simulink model "ConstantEnum"  (R2017b)
settings: Solver=FixedStepDiscrete  StartTime=0.0  StopTime=10.0  FixedStep=1.000000  RelTol=1e-3
model workspace (MAT data in the model file):
  ContractValidatorBlocksMap = containers.Map
  ContractValidatorBlocksMap.serialization.keys = {'DaysEnum/contract/validator', 'days/contract/validator'}
  ContractValidatorBlocksMap.serialization.values{1}.block = 'DaysEnum/contract/validator'
  ContractValidatorBlocksMap.serialization.values{1}.assumePorts = 0
  ContractValidatorBlocksMap.serialization.values{1}.guaranteePorts = 1
  ContractValidatorBlocksMap.serialization.values{1}.modeBlocksPorts = 0
  ContractValidatorBlocksMap.serialization.values{1}.portHandles.Inport = 64.0010986328
  ContractValidatorBlocksMap.serialization.values{1}.portHandles.Outport = 65.0003662109
  ContractValidatorBlocksMap.serialization.values{1}.portHandles.Enable = []
  ContractValidatorBlocksMap.serialization.values{1}.portHandles.Trigger = []
  ContractValidatorBlocksMap.serialization.values{1}.portHandles.State = []
  ContractValidatorBlocksMap.serialization.values{1}.portHandles.LConn = []
  ContractValidatorBlocksMap.serialization.values{1}.portHandles.RConn = []
  ContractValidatorBlocksMap.serialization.values{1}.portHandles.Ifaction = []
  ContractValidatorBlocksMap.serialization.values{1}.portHandles.Reset = []
  ContractValidatorBlocksMap.serialization.values{1}.portConnectivity(1).Type = '1'
  ContractValidatorBlocksMap.serialization.values{1}.portConnectivity(1).Position = [375 75]
  ContractValidatorBlocksMap.serialization.values{1}.portConnectivity(1).SrcBlock = 10.0003662109
  ContractValidatorBlocksMap.serialization.values{1}.portConnectivity(1).SrcPort = 0
  ContractValidatorBlocksMap.serialization.values{1}.portConnectivity(1).DstBlock = []
  ContractValidatorBlocksMap.serialization.values{1}.portConnectivity(1).DstPort = []
  ContractValidatorBlocksMap.serialization.values{1}.portConnectivity(2).Type = '1'
  ContractValidatorBlocksMap.serialization.values{1}.portConnectivity(2).Position = [505 75]
  ContractValidatorBlocksMap.serialization.values{1}.portConnectivity(2).SrcBlock = []
  ContractValidatorBlocksMap.serialization.values{1}.portConnectivity(2).SrcPort = []
  ContractValidatorBlocksMap.serialization.values{1}.portConnectivity(2).DstBlock = 35.0003662109
  ContractValidatorBlocksMap.serialization.values{1}.portConnectivity(2).DstPort = 0
  ContractValidatorBlocksMap.serialization.values{2}.block = 'days/contract/validator'
  ContractValidatorBlocksMap.serialization.values{2}.assumePorts = 0
  ContractValidatorBlocksMap.serialization.values{2}.guaranteePorts = 1
  ContractValidatorBlocksMap.serialization.values{2}.modeBlocksPorts = 0
  ContractValidatorBlocksMap.serialization.values{2}.portHandles.Inport = 174.00012207
  ContractValidatorBlocksMap.serialization.values{2}.portHandles.Outport = 168.000366211
  ContractValidatorBlocksMap.serialization.values{2}.portHandles.Enable = []
  ContractValidatorBlocksMap.serialization.values{2}.portHandles.Trigger = []
  ContractValidatorBlocksMap.serialization.values{2}.portHandles.State = []
  ContractValidatorBlocksMap.serialization.values{2}.portHandles.LConn = []
  ContractValidatorBlocksMap.serialization.values{2}.portHandles.RConn = []
  ContractValidatorBlocksMap.serialization.values{2}.portHandles.Ifaction = []
  ContractValidatorBlocksMap.serialization.values{2}.portHandles.Reset = []
  ContractValidatorBlocksMap.serialization.values{2}.portConnectivity(1).Type = '1'
  ContractValidatorBlocksMap.serialization.values{2}.portConnectivity(1).Position = [375 75]
  ContractValidatorBlocksMap.serialization.values{2}.portConnectivity(1).SrcBlock = 290.00012207
  ContractValidatorBlocksMap.serialization.values{2}.portConnectivity(1).SrcPort = 0
  ContractValidatorBlocksMap.serialization.values{2}.portConnectivity(1).DstBlock = []
  ContractValidatorBlocksMap.serialization.values{2}.portConnectivity(1).DstPort = []
  ContractValidatorBlocksMap.serialization.values{2}.portConnectivity(2).Type = '1'
  ContractValidatorBlocksMap.serialization.values{2}.portConnectivity(2).Position = [505 75]
  ContractValidatorBlocksMap.serialization.values{2}.portConnectivity(2).SrcBlock = []
  ContractValidatorBlocksMap.serialization.values{2}.portConnectivity(2).SrcPort = []
  ContractValidatorBlocksMap.serialization.values{2}.portConnectivity(2).DstBlock = 152.00012207
  ContractValidatorBlocksMap.serialization.values{2}.portConnectivity(2).DstPort = 0
  ContractValidatorBlocksMap.serialization.uniformity = 0
  ContractValidatorBlocksMap.serialization.keyType = 'char'
  ContractValidatorBlocksMap.serialization.valueType = 'any'
undefined symbols (not defined in the file): Days
libraries: simulink x3
settings Model: Creator=mudat  LastModifiedBy=hbourbou
settings CodeAppCC: StateflowObjectComments=on

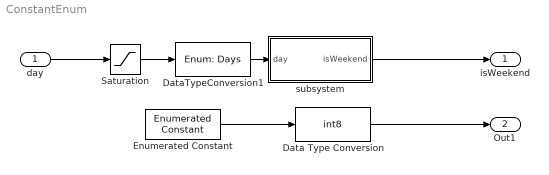
== system ConstantEnum ==
  day : Inport  OutMin=1  OutMax=7  OutDataTypeStr=uint8
  Data Type Conversion : DataTypeConversion  OutDataTypeStr=int8
  DataTypeConversion1 : DataTypeConversion  OutDataTypeStr=Enum: Days
  Enumerated Constant : simulink/Sources/Enumerated Constant  OutDataTypeStr=Enum: Days  Value=Days.Saturday  SampleTime=inf
      settings: SourceProductName=Simulink
  Saturation : Saturate  UpperLimit=7  LowerLimit=1  OutDataTypeStr=uint8
  subsystem : Subsystem
  isWeekend : Outport  OutDataTypeStr=boolean
  Out1 : Outport  Port=2
  wires:
  day/1 -> Saturation/1
  subsystem/1(isWeekend) -> isWeekend/1
  Enumerated Constant/1 -> Data Type Conversion/1
  Data Type Conversion/1 -> Out1/1
  Saturation/1 -> DataTypeConversion1/1
  DataTypeConversion1/1 -> subsystem/1(day)

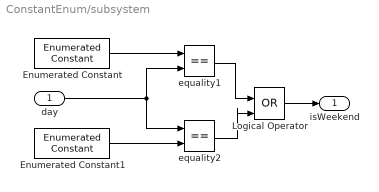
== system ConstantEnum/subsystem ==
  day : Inport  OutDataTypeStr=Enum: Days
  Enumerated Constant : simulink/Sources/Enumerated Constant  OutDataTypeStr=Enum: Days  Value=Days.Saturday  SampleTime=inf
      settings: SourceProductName=Simulink
  Enumerated Constant1 : simulink/Sources/Enumerated Constant  OutDataTypeStr=Enum: Days  Value=Days.Sunday  SampleTime=inf
      settings: SourceProductName=Simulink
  Logical Operator : Logic  Operator=OR  IconShape=distinctive  AllPortsSameDT=off  OutDataTypeStr=boolean
  equality1 : RelationalOperator  Operator===  OutDataTypeStr=boolean  RndMeth=Simplest
  equality2 : RelationalOperator  Operator===  OutDataTypeStr=boolean  RndMeth=Simplest
  isWeekend : Outport  OutDataTypeStr=boolean
  wires:
  Enumerated Constant/1 -> equality1/1
  Enumerated Constant1/1 -> equality2/2
  equality1/1 -> Logical Operator/1
  equality2/1 -> Logical Operator/2
  day/1 -> equality2/1, equality1/2
  Logical Operator/1 -> isWeekend/1
